simulink model "RP_VEX_V5_Gamepad_Control"  (R2019b)
settings: Solver=VariableStepAuto  StartTime=0.0  StopTime=inf  FixedStep=0.01  RelTol=1e-3  EnableMultiTasking=on
InitFcn:
  | RPInit
model workspace (MAT data in the model file):
  mapForSim.obsMap = [0 0 0 0 0 0 0 0 0 0 0 0 ... (25000 elements, 200x125)]
  mapForSim.scaleFactor = 25
  mapForSim.simMap = robotics.BinaryOccupancyGrid
  mapForSim.simMap.Grid = [1 1 1 1 1 1 1 1 1 1 1 1 ... (25000 elements, 200x125)]
  mapForSim.simMap.LayerName = "binaryLayer"
  mapForSim.simMap.Index = matlabshared.autonomous.internal.CircularBufferIndex
  mapForSim.simMap.Index.Head = [1 1]
  mapForSim.simMap.Index.Size = [200 125]
  mapForSim.simMap.Index.NewRegions = [0 0 0 0]
  mapForSim.simMap.Index.DropEntireMap = 0
  mapForSim.simMap.Index.DropTwoRegions = [0 0]
  mapForSim.simMap.Buffer = matlabshared.autonomous.internal.CircularBuffer
  mapForSim.simMap.Buffer.ConstVal = 0
  mapForSim.simMap.Buffer.DataType = 'logical'
  mapForSim.simMap.Buffer.Index = matlabshared.autonomous.internal.CircularBufferIndex
  mapForSim.simMap.Buffer.Index.Head = [1 1]
  mapForSim.simMap.Buffer.Index.Size = [200 125]
  mapForSim.simMap.Buffer.Index.NewRegions = [0 0 0 0]
  mapForSim.simMap.Buffer.Index.DropEntireMap = 0
  mapForSim.simMap.Buffer.Index.DropTwoRegions = [0 0]
  mapForSim.simMap.Buffer.Buffer = [1 1 1 1 1 1 1 1 1 1 1 1 ... (25000 elements, 200x125)]
  mapForSim.simMap.DefaultValueInternal = 0
  mapForSim.simMap.HasParent = 0
  mapForSim.simMap.Resolution = 25
  mapForSim.simMap.GridSize = [200 125]
  mapForSim.simMap.GridOriginInLocal = [0 0]
  mapForSim.simMap.LocalOriginInWorld = [0 0]
  mapForSim.simMap.Width = 5
  mapForSim.simMap.Height = 8
  mapForSim.simMap.LocalOriginInWorldInternal = [0 0]
  occGrid = robotics.BinaryOccupancyGrid
  occGrid.Grid = [1 1 1 1 1 1 1 1 1 1 1 1 ... (25000 elements, 200x125)]
  occGrid.LayerName = "binaryLayer"
  occGrid.Index = matlabshared.autonomous.internal.CircularBufferIndex
  occGrid.Index.Head = [1 1]
  occGrid.Index.Size = [200 125]
  occGrid.Index.NewRegions = [0 0 0 0]
  occGrid.Index.DropEntireMap = 0
  occGrid.Index.DropTwoRegions = [0 0]
  occGrid.Buffer = matlabshared.autonomous.internal.CircularBuffer
  occGrid.Buffer.ConstVal = 0
  occGrid.Buffer.DataType = 'logical'
  occGrid.Buffer.Index = matlabshared.autonomous.internal.CircularBufferIndex
  occGrid.Buffer.Index.Head = [1 1]
  occGrid.Buffer.Index.Size = [200 125]
  occGrid.Buffer.Index.NewRegions = [0 0 0 0]
  occGrid.Buffer.Index.DropEntireMap = 0
  occGrid.Buffer.Index.DropTwoRegions = [0 0]
  occGrid.Buffer.Buffer = [1 1 1 1 1 1 1 1 1 1 1 1 ... (25000 elements, 200x125)]
  occGrid.DefaultValueInternal = 0
  occGrid.HasParent = 0
  occGrid.Resolution = 25
  occGrid.GridSize = [200 125]
  occGrid.GridOriginInLocal = [0 0]
  occGrid.LocalOriginInWorld = [0 0]
  occGrid.Width = 5
  occGrid.Height = 8
  occGrid.LocalOriginInWorldInternal = [0 0]
undefined symbols (not defined in the file): FloorSurface, Ref, RobotSurface, X, Y, Z
libraries: sm_lib x21, RP_Simulator_Components x12, nesl_utility x11, simulink x3, vexv5lib x3, RoboticsPlayground x2, vexcommonlib x1, vrlib x1
(part 1 of 2)
settings Model: EnablePacing=on  ExtModeTrigDuration=25  Creator=scastro  LastModifiedBy=josea
settings SolverCC: AlgebraicLoopSolver=LineSearch
settings DataIOCC: LimitDataPoints=on  ReturnWorkspaceOutputs=off
settings OptimizationCC: PassReuseOutputArgsAs=Individual arguments  MaxStackSize=64  EfficientTunableParamExpr=on
settings DebuggingCC: ParameterTunabilityLossMsg=error  UnconnectedLineMsg=none  AllowSymbolicDim=off  SFUnexpectedBacktrackingDiag=warning  SFNoUnconditionalDefaultTransitionDiag=warning  SFExecutionAtInitializationDiag=none  ArithmeticOperatorsInVariantConditions=warning
settings HardwareCC: ProdBitPerPointer=32  ProdBitPerSizeT=32  ProdBitPerPtrDiffT=32  ProdLargestAtomicInteger=Long  ProdLargestAtomicFloat=Double  ProdWordSize=32  ProdHWDeviceType=ARM Compatible->ARM Cortex
settings SFSimCC: SimUseLocalCustomCode=off  MATLABDynamicMemAlloc=off  CustomCodeUndefinedFunction=UseInterfaceOnly
settings RTWCC: SystemTargetFile=ert.tlc  HardwareBoard=VEX V5 Robot Brain  TLCOptions="-aInlineSetEventsForThisBaseRateFcn=TLC_FALSE -aSuppressMultiTaskScheduler=TLC_FALSE  -aRateBasedStepFcn=0"  TemplateMakefile=ert_default_tmf  GenerateReport=on  RTWUseLocalCustomCode=off  Toolchain=GNU Tools for ARM Embedded Processors  IncludeHyperlinkInReport=on  LaunchReport=on  GenerateTraceInfo=on  GenerateTraceReport=on  GenerateTraceReportSl=on  GenerateTraceReportSf=on  GenerateTraceReportEml=on
settings CodeAppCC: ForceParamTrailComments=on  IgnoreCustomStorageClasses=off  OperatorAnnotations=on  SimulinkDataObjDesc=on  SFDataObjDesc=on  InsertBlockDesc=on
settings ERTTargetCC: ExtModeStaticAllocSize=2048
settings ConfigComp: CovMetricSettings=dw  CovHtmlReporting=on  CovSaveCumulativeToWorkspaceVar=on  CovSaveSingleToWorkspaceVar=on  CovExternalEMLEnable=off  CovSFcnEnable=off
settings SimscapeCC: SimscapeNominalValues="[{\"value\":\"10\",\"unit\":\"V\"},{\"value\":\"1\",\"unit\":\"A\"},{\"value\":\"10\",\"unit\":\"N*m\"},{\"value\":\"10\",\"unit\":\"bar\"},{\"value\":\"100\",\"unit\":\"kJ/kg\"},{\"value\":\"1\",\"unit\":\"kW\"},{\"value\":\"300\",\"unit\":\"K\"},{\"value\":\"100\",\"unit\":\"cm^3/s\"},{\"value\":\"1\",\"unit\":\"kN\"},{\"value\":\"1\",\"unit\":\"g/cm^3\"},{\"value\":\"1\",\"unit\":\"l\"},{\"value\":\"1\",\"unit\":\"cm^2\"},{\"value\":\"60\",\"unit\":\"Hz\"}]"  SimscapeLogDataHistory=10000
settings ConfigurationSet: Description=SimMechanics 2G
settings DiagnosticsConfigSet: SimMechanicsRigidlyBoundBlock=none
settings ExplorerConfigSet: InternalSimMechanicsExplorerSettings="<ExplorerConfiguration><canonicalview>default</canonicalview><AnimationSetting><BasePlaybackSpeed>1.0</BasePlaybackSpeed><PlaybackSpeedFactor>1.0</PlaybackSpeedFactor></AnimationSetting><TilePanel><TileInfo><Tiles Columns=\"2\" Count=\"3\" Rows=\"2\"><Column Weight=\"0.5\"/><Column Weight=\"0.5\"/><Row Weight=\"0.5558\"/><Row Weight=\"0.4442\"/><Tile Height=\"1\" Width=\"2\" X=\"0\" Y=\"0\"/><Tile Height=\"1\" Width=\"1\" X=\"0\" Y=\"1\"/><Tile Height=\"1\" Width=\"1\" X=\"1\" Y=\"1\"/></Tiles></TileInfo><SceneInfo><SceneViewer><BGColor><R>0.60000002384185791</R><G>0.60000002384185791</G><B>0.60000002384185791</B></BGColor><Camera><DoPerspective>off</DoPerspective><Position><X>3.77812343469301437</X><Y>-3.77812335288872925</Y><Z>3.7781233369241094</Z></Position><Center><X>-2.07139932301910341e-08</X><Y>1.02518278512960765e-07</Y><Z>-1.18482898008922e-07</Z></Center><Up><X>-0.408248290463863073</X><Y>0.408248290463863073</Y><Z>0.816496580927726145</Z></Up><ViewLimDist>1</ViewLimDist><YLim>2.86778095960617074</YLim><XLim>6.75102172519388599</XLim></Camera></SceneViewer><SceneViewer><BGColor><R>0.60000002384185791</R><G>0.60000002384185791</G><B>0.60000002384185791</B></BGColor><Camera><DoPerspective>on</DoPerspective><Position><X>0.025687663764123736</X><Y>0.399310018201750161</Y><Z>0.453907703599162216</Z></Position><Center><X>0.541332794341274459</X><Y>-0.386267680610761999</Y><Z>0.111887560273493503</Z></Center><Up><X>0.187679478974392022</X><Y>-0.285926899071094254</Y><Z>0.939692620785908428</Z></Up><ViewLimDist>1</ViewLimDist><YLim>0.466307658154998583</YLim><XLim>0.683848507606772515</XLim></Camera></SceneViewer><SceneViewer><BGColor><R>0.60000002384185791</R><G>0.60000002384185791</G><B>0.60000002384185791</B></BGColor><Camera><DoPerspective>off</DoPerspective><Position><X>-0.018234885227883621</X><Y>-0.0300165861003731764</Y><Z>37.6782594368875863</Z></Position><Center><X>-0.018234885227883621</X><Y>-0.0300165861003731764</Y><Z>0.069999846435872648</Z></Center><Up><X>0</X><Y>1</Y><Z>-0</Z></Up><ViewLimDist>1</ViewLimDist><YLim>5.44437616630040022</YLim><XLim>7.98427486888250648</XLim></Camera></SceneViewer></SceneInfo></TilePanel><MechEditorPanel><Cameras><Camera><Id>Camera1</Id><Value><Name>RobotView</Name><NativeCamera><PositionTrackingFeature>Obstacle_Environment.Robot.Body.RobotCamera.F</PositionTrackingFeature><CenterTrackingFeature>Obstacle_Environment.Robot.Body.RobotCamera.F</CenterTrackingFeature><UpVectorTrackingFeature>Obstacle_Environment.Robot.Body.RobotCamera.F</UpVectorTrackingFeature><CenterTrackingOrigin>off</CenterTrackingOrigin><CenterTrackingDirection>+X</CenterTrackingDirection><UpVectorTrackingDirection>+Z</UpVectorTrackingDirection></NativeCamera></Value></Camera></Cameras><GfxPanelCameraMap><MapElement CameraMLId=\"Camera1\" GfxPanelIndex=\"1\"/></GfxPanelCameraMap><VideoCreator><PlaybackSpeedRatio>1.0</PlaybackSpeedRatio><FrameRate>30</FrameRate><VideoFormat>Motion JPEG AVI</VideoFormat><FrameSize>auto</FrameSize></VideoCreator></MechEditorPanel></ExplorerConfiguration>"

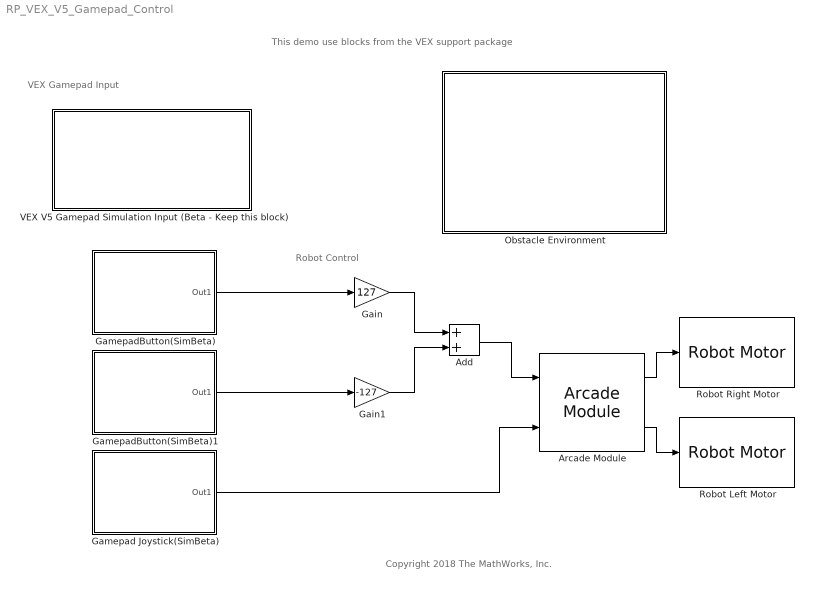
== system RP_VEX_V5_Gamepad_Control ==
  note: VEX Gamepad Input
  note: Robot Control
  note: Copyright 2018 The MathWorks, Inc.
  note: This demo use blocks from the VEX support package
  Add : Sum
  Arcade Module : vexcommonlib/Arcade Module  BlockPlatform=vexarmcortex
      settings: SourceProductName=Simulink Coder Support Package for ARM Cortex-based VEX Microcontroller  SourceProductBaseCode=EC_VEX_MICRO
  Gain : Gain  Gain=127
  Gain1 : Gain  Gain=-127
  Gamepad Joystick(SimBeta) : Subsystem  mask(Gamepad Joystick (Simulation Beta)){joystickType=Master, chan=1, SampleTime=0.02}
      mask prompts: joystickType "Joystick Type:"; chan "Analog Channel (1 to 4):"; SampleTime "Sample time:"
      mask help:
      | Read the value from one of the control axis of the analog joysticks on the VEX® gamepad(V5 controller).
      |
      | The output ranges from -128 to 127 and 0 indicates that the joystick has not been displaced.
      |
      | Use Gamepad Type to configure the gamepad to operate in Master or Partner mode.
      |
      | Use the Analog Channel drop-down to specify the control axis of the joystick on the VEX® gamepad from which you would like to read an analog signal. The Analog Channel number must match the labels on the gamepad.
      mask init:
      | chan = get_param(gcb, 'chan');
      | joyIdStr = get_param(gcb,'joystickType');
      | if strcmp(joyIdStr,'Partner')
      |     joyId='2';
      | else
      |     joyId='1';
      | end
      | 
      | set_param([gcb '/GamepadJoysticks'],'GoToTag',['simGamepadJoysticks_' joyId]);
      | 
      | if chan == '2' 
      |     md = 'icon=imread(fullfile(codertarget.vexv5.internal.getSpPkgRootDir, ''resources'', ''JoystickAnalog2.png''));icon(1:350,1:772,:)=imread(''vexv5GamepadSimInput.PNG'');image(icon)';
      |     set_param([gcb '/Channel'],'Value',chan);
      | elseif chan == '1'
      |     md = 'icon=imread(fullfile(codertarget.vexv5.internal.getSpPkgRootDir, ''resources'', ''JoystickAnalog1.png''));icon(1:350,1:772,:)=imread(''vexv5GamepadSimInput.PNG'');image(icon)';   
      |     set_param([gcb '/Channel'],'Value',chan);
      | elseif chan == '4'
      |     md = 'icon=imread(fullfile(codertarget.vexv5.internal.getSpPkgRootDir, ''resources'', ''JoystickAnalog4.png''));icon(1:350,1:772,:)=imread(''vexv5GamepadSimInput.PNG'');image(icon)';   
      |     set_param([gcb '/Channel'],'Value',chan);
      | elseif chan == '3'
      |     md = 'icon=imread(fullfile(codertarget.vexv5.internal.getSpPkgRootDir, ''resources'', ''JoystickAnalog3.png''));icon(1:350,1:772,:)=imread(''vexv5GamepadSimInput.PNG'');image(icon)';    
      |     set_param([gcb '/Channel'],'Value',chan);
      | end
      | blPosition = get_param(gcb, 'Position');
      | textSize = get_param(gcb, 'fontSize');
      | if textSize==-1
      |     textSize = get_param(bdroot, 'DefaultBlockFontSize');
      | end
      | md = codertarget.vexv5.internal.writeVEXOnMask(gcb, md);
      | set_param(gcb, 'MaskDisplay', md);
      mask TypeOptions joystickType: Gamepad Joystick/joystickType
      mask TypeOptions chan: Gamepad Joystick/chan
      mask TypeOptions SampleTime: Gamepad Joystick/SampleTime
      mask Display:
      | icon=imread(fullfile(codertarget.vexv5.internal.getSpPkgRootDir, 'resources', 'JoystickAnalog1.png'));icon(1:350,1:772,:)=imread('vexv5GamepadSimInput.PNG');image(icon)
      | patch([0.65, 0.65, 1, 1], [0.85, 1, 1, 0.85], [1, 1, 1]);
      | color('blue');
      | text(1, 1, 'VEX V5', 'horizontalAlignment', 'right', 'verticalAlignment','top');
  GamepadButton(SimBeta) : Subsystem  mask(Gamepad Button (Simulation Beta)){joystickType=Master, chan=UP, SampleTime=0.02}
      mask prompts: joystickType "Joystick Type:"; chan "Button:"; SampleTime "Sample time:"
      mask help:
      | Read the logical value of the selected button from the VEX® gamepad(V5 controller).
      |
      | The  output is 1 while the button is in pressed state and 0 while the button is in release state.
      |
      | Use Gamepad Type to configure the gamepad to operate in Master or Partner mode.
      | Use the Button drop-down to specify the button on the VEX® gamepad from which you would like to read a digital signal. The Button must match the labels on the gamepad.
      mask init:
      | chan = get_param(gcb, 'chan');
      | joyIdStr = get_param(gcb,'joystickType');
      | if strcmp(joyIdStr,'Partner')
      |     joyId='2';
      | else
      |     joyId='1';
      | end
      | set_param([gcb '/GamepadButtons'],'GoToTag',['simGamepadButtons_' joyId]);
      | 
      | if strcmp(chan,'L2') 
      |     md = 'icon=imread(fullfile(codertarget.vexv5.internal.getSpPkgRootDir, ''resources'', ''JoystickDigitalButton_L2.png''));icon(1:31,1:60,:)=imread(''vexv5GamepadSimInput2.PNG'');image(icon)';
      |     set_param([gcb '/Channel'],'Value','10');
      | elseif strcmp(chan,'L1') 
      |     md = 'icon=imread(fullfile(codertarget.vexv5.internal.getSpPkgRootDir, ''resources'', ''JoystickDigitalButton_L1.png''));icon(1:31,1:60,:)=imread(''vexv5GamepadSimInput2.PNG'');image(icon)';
      |     set_param([gcb '/Channel'],'Value','9');
      | elseif strcmp(chan,'R2') 
      |     md = 'icon=imread(fullfile(codertarget.vexv5.internal.getSpPkgRootDir, ''resources'', ''JoystickDigitalButton_R2.png''));icon(1:31,1:60,:)=imread(''vexv5GamepadSimInput2.PNG'');image(icon)';
      |     set_param([gcb '/Channel'],'Value','12');
      | elseif strcmp(chan,'R1') 
      |     md = 'icon=imread(fullfile(codertarget.vexv5.internal.getSpPkgRootDir, ''resources'', ''JoystickDigitalButton_R1.png''));icon(1:31,1:60,:)=imread(''vexv5GamepadSimInput2.PNG'');image(icon)';
      |     set_param([gcb '/Channel'],'Value','11');
      | elseif strcmp(chan,'DOWN') 
      |      md = 'icon=imread(fullfile(codertarget.vexv5.internal.getSpPkgRootDir, ''resources'', ''JoystickDigitalDown.png''));icon(1:31,1:60,:)=imread(''vexv5GamepadSimInput2.PNG'');image(icon)';
      |      set_param([gcb '/Channel'],'Value','2');
      | elseif strcmp(chan,'UP') 
      |     md = 'icon=imread(fullfile(codertarget.vexv5.internal.getSpPkgRootDir, ''resources'', ''JoystickDigitalUp.png''));icon(1:31,1:60,:)=imread(''vexv5GamepadSimInput2.PNG'');image(icon)';
      |     set_param([gcb '/Channel'],'Value','1');
      | elseif strcmp(chan,'LEFT') 
      |     md = 'icon=imread(fullfile(codertarget.vexv5.internal.getSpPkgRootDir, ''resources'', ''JoystickDigitalLeft.png''));icon(1:31,1:60,:)=imread(''vexv5GamepadSimInput2.PNG'');image(icon)';
      |     set_param([gcb '/Channel'],'Value','3');
      | elseif strcmp(chan,'RIGHT') 
      |     md = 'icon=imread(fullfile(codertarget.vexv5.internal.getSpPkgRootDir, ''resources'', ''JoystickDigitalRight.png''));icon(1:31,1:60,:)=imread(''vexv5GamepadSimInput2.PNG'');image(icon)';
      |     set_param([gcb '/Channel'],'Value','4');
      | elseif chan == 'B' 
      |     md = 'icon=imread(fullfile(codertarget.vexv5.internal.getSpPkgRootDir, ''resources'', ''JoystickDigitalButton_B.png''));icon(1:31,1:60,:)=imread(''vexv5GamepadSimInput2.PNG'');image(icon)';
      |     set_param([gcb '/Channel'],'Value','6');
      | elseif chan == 'X' 
      |     md = 'icon=imread(fullfile(codertarget.vexv5.internal.getSpPkgRootDir, ''resources'', ''JoystickDigitalButton_X.png''));icon(1:31,1:60,:)=imread(''vexv5GamepadSimInput2.PNG'');image(icon)';
      |     set_param([gcb '/Channel'],'Value','7');
      | elseif chan == 'Y' 
      |     md = 'icon=imread(fullfile(codertarget.vexv5.internal.getSpPkgRootDir, ''resources'', ''JoystickDigitalButton_Y.png''));icon(1:31,1:60,:)=imread(''vexv5GamepadSimInput2.PNG'');image(icon)';
      |     set_param([gcb '/Channel'],'Value','8');
      | elseif chan == 'A' 
      |     md = 'icon=imread(fullfile(codertarget.vexv5.internal.getSpPkgRootDir, ''resources'', ''JoystickDigitalButton_A.png''));icon(1:31,1:60,:)=imread(''vexv5GamepadSimInput2.PNG'');image(icon)';
      |     set_param([gcb '/Channel'],'Value','5');
      | end
      | 
      | md = codertarget.vexv5.internal.writeVEXOnMask(gcb, md);
      | set_param(gcb, 'MaskDisplay', md);
      mask TypeOptions joystickType: Gamepad Button/joystickType
      mask TypeOptions chan: Gamepad Button/chan
      mask TypeOptions SampleTime: Gamepad Button/SampleTime
      mask Display:
      | icon=imread(fullfile(codertarget.vexv5.internal.getSpPkgRootDir, 'resources', 'JoystickDigitalUp.png'));icon(1:31,1:60,:)=imread('vexv5GamepadSimInput2.PNG');image(icon)
      | patch([0.65, 0.65, 1, 1], [0.85, 1, 1, 0.85], [1, 1, 1]);
      | color('blue');
      | text(1, 1, 'VEX V5', 'horizontalAlignment', 'right', 'verticalAlignment','top');
  GamepadButton(SimBeta)1 : Subsystem  mask(Gamepad Button (Simulation Beta)){joystickType=Master, chan=DOWN, SampleTime=0.02}
      mask prompts: joystickType "Joystick Type:"; chan "Button:"; SampleTime "Sample time:"
      mask help:
      | Read the logical value of the selected button from the VEX® gamepad(V5 controller).
      |
      | The  output is 1 while the button is in pressed state and 0 while the button is in release state.
      |
      | Use Gamepad Type to configure the gamepad to operate in Master or Partner mode.
      | Use the Button drop-down to specify the button on the VEX® gamepad from which you would like to read a digital signal. The Button must match the labels on the gamepad.
      mask init: same as RP_VEX_V5_Gamepad_Control/GamepadButton(SimBeta)
      mask TypeOptions joystickType: Gamepad Button/joystickType
      mask TypeOptions chan: Gamepad Button/chan
      mask TypeOptions SampleTime: Gamepad Button/SampleTime
      mask Display:
      | icon=imread(fullfile(codertarget.vexv5.internal.getSpPkgRootDir, 'resources', 'JoystickDigitalDown.png'));icon(1:31,1:60,:)=imread('vexv5GamepadSimInput2.PNG');image(icon)
      | patch([0.65, 0.65, 1, 1], [0.85, 1, 1, 0.85], [1, 1, 1]);
      | color('blue');
      | text(1, 1, 'VEX V5', 'horizontalAlignment', 'right', 'verticalAlignment','top');
  Obstacle Environment : Subsystem  mask(RP Obstacle Environment){obs1=on, obsPose1=[0.14251      3.2953], obsWidth1=4.0293, obsLength1=0.31625, obs2=on, obsPose2=[1.8233    -0.44119], obsWidth2=0.24597, obsLength2=5.7042, obs3=on, obsPose3=[-0.33772     -3.1938], obsWidth3=3.3734, obsLength3=0.55051, obs4=on, obsPose4=[-0.43729    -0.97413], obsWidth4=3.1274, obsLength4=0.37482, obs5=off, obsPose5=[1.6535    -0.67545], obsWidth5=0.39824, obsLength5=0.71449, obs6=off, obsPose6=[3.1293     -1.6301], obsWidth6=0.60322, obsLength6=0.47438, obs7=off, obsPose7=[2 2], obsWidth7=0.8, obsLength7=0.4, obs8=off, obsPose8=[2 2], obsWidth8=0.8, obsLength8=0.4, obs9=off, obsPose9=[2 2], obsWidth9=0.8, obsLength9=0.4, obs10=off, obsPose10=[2 2], obsWidth10=0.8, obsLength10=0.4, arenaLength=5, arenaWidth=8, robotId=1, wheelBase=0.5, wheelRadius=0.1, robotColor=[0 0 0.5], startPose=[-1.4 0]}
      mask prompts: obs1 "Enable"; obsPose1 "Position X Y [m]"; obsWidth1 "Width [m]"; obsLength1 "Length [m]"; obs2 "Enable"; obsPose2 "Position X Y [m]"; obsWidth2 "Width [m]"; obsLength2 "Length [m]"; obs3 "Enable"; obsPose3 "Position X Y [m]"; obsWidth3 "Width [m]"; obsLength3 "Length [m]"; obs4 "Enable"; obsPose4 "Position X Y [m]"; obsWidth4 "Width [m]"; obsLength4 "Length [m]"; obs5 "Enable"; obsPose5 "Position X Y [m]"; obsWidth5 "Width [m]"; obsLength5 "Length [m]"; obs6 "Enable"; obsPose6 "Position X Y [m]"; obsWidth6 "Width [m]"; obsLength6 "Length [m]"; obs7 "Enable"; obsPose7 "Position X Y [m]"; obsWidth7 "Width [m]"; obsLength7 "Length [m]"; obs8 "Enable"; obsPose8 "Position X Y [m]"; obsWidth8 "Width [m]"; obsLength8 "Length [m]"; obs9 "Enable"; obsPose9 "Position X Y [m]"; obsWidth9 "Width [m]"; obsLength9 "Length [m]"; obs10 "Enable"; obsPose10 "Position X Y [m]"; obsWidth10 "Width [m]"; obsLength10 "Length [m]"; arenaLength "Length [m]"; arenaWidth "Width [m]"; robotId "Robot ID"; wheelBase "Distance between wheels [m]"; wheelRadius "Wheel radius [m]"; robotColor "Color [R G B]"; startPose "Initial Position X Y [m]"
      mask help:
      | This block contains a virtual environment for a single robot to interact with walls, obstacles and objects. Sensors implemented in the Robotics Playground library can be used to obtain environment information and actuators to interact with the robot behavior.
      |
      | Motor mapping for the robot is as follows:
      |
      | Motor 1 -> Left wheel motor torque
      | Motor 2 -> Right wheel motor torque
      settings: CopyFcn=|
      | set_param(gcs,'InitFcn','RPInit');
      | set_param(gcs,'Solver','ode23t');
      | set_param(gcs, 'EnablePacing', 'on')
      | set_param(gcs, 'PacingRate', 1)
      mask Help: web('obstacle_arena.htm')
      mask Callback obs1: commentObstacles(gcb)
      mask Callback obs2: commentObstacles(gcb)
      mask Callback obs3: commentObstacles(gcb)
      mask Callback obs4: commentObstacles(gcb)
      mask Callback obs5: commentObstacles(gcb)
      mask Callback obs6: commentObstacles(gcb)
      mask Callback obs7: commentObstacles(gcb)
      mask Callback obs8: commentObstacles(gcb)
      mask Callback obs9: commentObstacles(gcb)
      mask Callback obs10: commentObstacles(gcb)
      mask DialogControl obsT Prompt: Obstacle settings
      mask DialogControl Container19 Prompt: Set Obstacles Interactively
      mask DialogControl Control2 Prompt: Set Obstacles
      mask DialogControl Control2 Callback: setObstaclesUI(gcb)
      mask DialogControl Control3 Prompt: Disable all obstacles
      mask DialogControl Control3 Callback: disableObstacles(gcb)
      mask DialogControl Container21 Prompt: Obstacle Details
      mask DialogControl obsc1 Prompt: Obstacle 1
      mask DialogControl obsc2 Prompt: Obstacle 2
      mask DialogControl obsc3 Prompt: Obstacle 3
      mask DialogControl obsc4 Prompt: Obstacle 4
      mask DialogControl obsc5 Prompt: Obstacle 5
      mask DialogControl obsc6 Prompt: Obstacle 6
      mask DialogControl obsc7 Prompt: Obstacle 7
      mask DialogControl obsc8 Prompt: Obstacle 8
      mask DialogControl obsc9 Prompt: Obstacle 9
      mask DialogControl obsc10 Prompt: Obstacle 10
      mask DialogControl Container6 Prompt: Arena settings
      mask DialogControl Container4 Prompt: Robot settings
      mask Display:
      | color('white');
      | plot([100,100,100,100]*1,[100,100,100,100]*1);
      | plot([100,100,100,100]*0,[100,100,100,100]*0);
      | image('ObstacleEnv.PNG')
      | color('blue');
      | id=eval(get_param(gcb,'robotId'));
      | text(99, 92, ['Robot ID: ' num2str(id)], 'horizontalAlignment', 'right');
  Robot Left Motor : RoboticsPlayground/Basic Sensors and Actuators/Robot Motor  robotId=1  motorChoice=1
      settings: SourceProductName=Robotics Playground
  Robot Right Motor : RoboticsPlayground/Basic Sensors and Actuators/Robot Motor  robotId=1  motorChoice=2
      settings: SourceProductName=Robotics Playground
  VEX V5 Gamepad Simulation Input (Beta - Keep this block) : Subsystem  mask(VEX V5 Gamepad Simulation Input){gamepadChoice=1- Master}
      mask prompts: gamepadChoice "Gamepad Selection"
      mask help: This blocks uses the input from the VEX V5 Gamepad for desktop simulations. A V5 gamepad must be connected directly to the computer using a USB cable.
      mask init:
      | joyIdStr = get_param(gcb,'gamepadChoice');
      | if strcmp(joyIdStr,'2- Partner')
      |     joyId='2';
      | else
      |     joyId='1';
      | end
      | set_param([gcb '/Joystick Input'],'joyid',joyId);
      | set_param([gcb '/GamepadJoysticks'],'GoToTag',['simGamepadJoysticks_' joyId]);
      | set_param([gcb '/GamepadButtons'],'GoToTag',['simGamepadButtons_' joyId]);
      mask TypeOptions gamepadChoice: 1- Master | 2- Partner
      mask Display: image('vexv5GamepadSimInput.PNG')
  wires:
  Arcade Module/1 -> Robot Right Motor/1
  Arcade Module/2 -> Robot Left Motor/1
  Add/1 -> Arcade Module/1
  Gamepad Joystick(SimBeta)/1(Out1) -> Arcade Module/2
  GamepadButton(SimBeta)/1(Out1) -> Gain/1
  GamepadButton(SimBeta)1/1(Out1) -> Gain1/1
  Gain/1 -> Add/1
  Gain1/1 -> Add/2

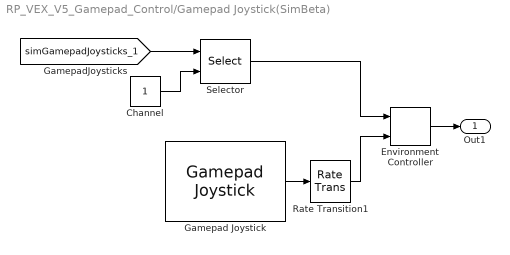
== system RP_VEX_V5_Gamepad_Control/Gamepad Joystick(SimBeta) ==
  Channel : Constant
  Environment Controller : simulink/Signal Routing/Environment Controller
      settings: SourceProductName=Simulink  SourceProductBaseCode=SL
  Gamepad Joystick : vexv5lib/Gamepad/Gamepad Joystick  joystickType=Master  chan=1  SampleTime=SampleTime
      settings: SourceProductName=Simulink Coder Support Package for VEX EDR V5 Robot Brain  SourceProductBaseCode=VEXV5
  Rate Transition1 : RateTransition
  Selector : Selector  InputPortWidth=4  IndexOptions=Index vector (port)  Indices=[1 3]  OutputSizes=1
  Out1 : Outport
  wires:
  Rate Transition1/1 -> Environment Controller/2
  Selector/1 -> Environment Controller/1
  Channel/1 -> Selector/2
  [simGamepadJoysticks_1] -> Selector/1
  Environment Controller/1 -> Out1/1
  Gamepad Joystick/1 -> Rate Transition1/1

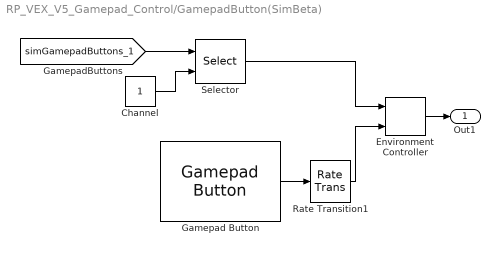
== system RP_VEX_V5_Gamepad_Control/GamepadButton(SimBeta) ==
  Channel : Constant
  Environment Controller : simulink/Signal Routing/Environment Controller
      settings: SourceProductName=Simulink  SourceProductBaseCode=SL
  Gamepad Button : vexv5lib/Gamepad/Gamepad Button  joystickType=Master  chan=UP  SampleTime=SampleTime
      settings: SourceProductName=Simulink Coder Support Package for VEX EDR V5 Robot Brain  SourceProductBaseCode=VEXV5
  Rate Transition1 : RateTransition
  Selector : Selector  InputPortWidth=12  IndexOptions=Index vector (port)  Indices=[1 3]  OutputSizes=1
  Out1 : Outport
  wires:
  Rate Transition1/1 -> Environment Controller/2
  Gamepad Button/1 -> Rate Transition1/1
  Environment Controller/1 -> Out1/1
  [simGamepadButtons_1] -> Selector/1
  Channel/1 -> Selector/2
  Selector/1 -> Environment Controller/1

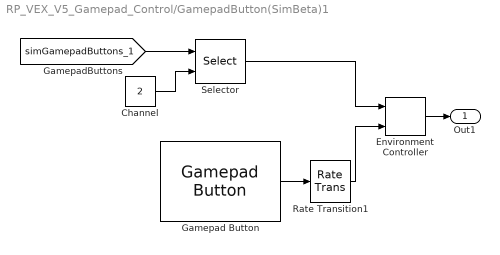
== system RP_VEX_V5_Gamepad_Control/GamepadButton(SimBeta)1 ==
  Channel : Constant  Value=2
  Environment Controller : simulink/Signal Routing/Environment Controller
      settings: SourceProductName=Simulink  SourceProductBaseCode=SL
  Gamepad Button : vexv5lib/Gamepad/Gamepad Button  joystickType=Master  chan=DOWN  SampleTime=SampleTime
      settings: SourceProductName=Simulink Coder Support Package for VEX EDR V5 Robot Brain  SourceProductBaseCode=VEXV5
  Rate Transition1 : RateTransition
  Selector : Selector  InputPortWidth=12  IndexOptions=Index vector (port)  Indices=[1 3]  OutputSizes=1
  Out1 : Outport
  wires:
  Selector/1 -> Environment Controller/1
  Channel/1 -> Selector/2
  [simGamepadButtons_1] -> Selector/1
  Environment Controller/1 -> Out1/1
  Gamepad Button/1 -> Rate Transition1/1
  Rate Transition1/1 -> Environment Controller/2

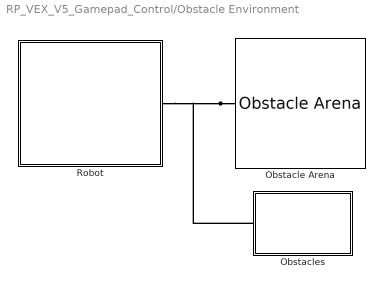
== system RP_VEX_V5_Gamepad_Control/Obstacle Environment ==
  Obstacle Arena : RP_Simulator_Components/Obstacle Arena  length=arenaLength  width=arenaWidth  robotRadius=wheelBase/2
  Obstacles : Subsystem
  Robot : Subsystem  AncestorBlock=RP_Simulator_Components/Contact Tank Robot  mask(RP Contact Tank Robot){robotId=robotId, wheelRadius=wheelRadius, wheelBase=wheelBase, wheelThickness=0.025, chassisThickness=0.05, startPose=startPose, choice=off, sensorTs=0.05, wheelMass=0.2, chassisMass=0.5, maxWheelTorque=1, floorSize=[arenaLength arenaWidth], wheelColor=[0.25 0.25 0.25], chassisColor=robotColor}
      mask prompts: robotId "Robot ID"; wheelRadius "Wheel Radius [m]"; wheelBase "Wheelbase [m]"; wheelThickness "Wheel Thickness [m]"; chassisThickness "Chassis Thickness [m]"; startPose "Start Position [m]"; choice "Reverse Start Position"; sensorTs "Sensor sample time [s]"; wheelMass "Wheel Mass [kg]"; chassisMass "Chassis Mass [kg]"; maxWheelTorque "Maximum wheel torque [N*m]"; floorSize "Floor Dimensions [m]"; wheelColor "Wheel Color"; chassisColor "Chassis Color"
      mask help:
      | This robot implements contact between the robot wheels and the floor of an arena. The stck-slip friction implemented using contact force libraries makes the robot behavior more realistic. The inputs to the robot are now motor torque, which is set using the Robotics Playground Motor blocks. The motor mappings are as follows:
      |
      | Motor 1 -> Left wheel motor torque
      | Motor 2 -> Right wheel motor torque
      mask init:
      | block=gcb;
      | ID=num2str(eval(get_param(block,'robotId')));
      | 
      | set_param([block '/motor1t'],'GotoTag',['R' ID 'motor1t']);
      | set_param([block '/motor2t'],'GotoTag',['R' ID 'motor2t']);
      | set_param([block '/motor1q'],'GotoTag',['R' ID 'motor1q']);
      | set_param([block '/motor1w'],'GotoTag',['R' ID 'motor1w']);
      | set_param([block '/motor2q'],'GotoTag',['R' ID 'motor2q']);
      | set_param([block '/motor2w'],'GotoTag',['R' ID 'motor2w']);
      | set_param([block '/xPose'],'GotoTag',['R' ID 'xPose']);
      | set_param([block '/yPose'],'GotoTag',['R' ID 'yPose']);
      | set_param([block '/tPose'],'GotoTag',['R' ID 'tPose']);
      | set_param([block '/tRate'],'GotoTag',['R' ID 'tRate']);
      | set_param([block '/tAngle'],'GotoTag',['R' ID 'tAngle']);
      | 
      | % Add sensor visuals
      | 
      | addSensors(block,eval(ID));
      mask DialogControl KinContainer Prompt: Kinematics
      mask DialogControl DynamicsContainer Prompt: Dynamics
      mask DialogControl AppearanceContainer Prompt: Appearance
      mask Display:
      | image('discRobot.PNG')
      | port_label('Rconn',1,'RP-Bus')
  connections:
  Obstacle Arena/LConn1 -- Robot/RConn1 -- Obstacles/LConn1

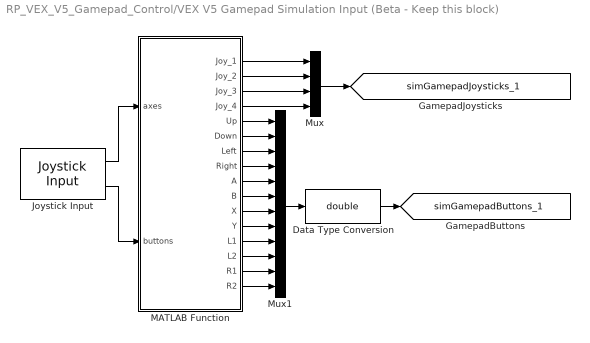
== system RP_VEX_V5_Gamepad_Control/VEX V5 Gamepad Simulation Input (Beta - Keep this block) ==
  Data Type Conversion : DataTypeConversion  OutDataTypeStr=double
  Joystick Input : vrlib/Joystick Input  joyid=1  adjustports=on  forcefeed=off
      settings: SourceProductName=Simulink
  MATLAB Function : MATLAB Function  TreatAsAtomicUnit=on
  Mux : Mux
  Mux1 : Mux  Inputs=12
  tag scope: simGamepadButtons_1=global, simGamepadJoysticks_1=global
  wires:
  Joystick Input/1 -> MATLAB Function/1(axes)
  Joystick Input/2 -> MATLAB Function/2(buttons)
  MATLAB Function/16(R2) -> Mux1/12
  MATLAB Function/15(R1) -> Mux1/11
  MATLAB Function/14(L2) -> Mux1/10
  MATLAB Function/13(L1) -> Mux1/9
  MATLAB Function/12(Y) -> Mux1/8
  MATLAB Function/11(X) -> Mux1/7
  MATLAB Function/10(B) -> Mux1/6
  MATLAB Function/9(A) -> Mux1/5
  MATLAB Function/8(Right) -> Mux1/4
  MATLAB Function/7(Left) -> Mux1/3
  MATLAB Function/6(Down) -> Mux1/2
  MATLAB Function/5(Up) -> Mux1/1
  Mux/1 -> [simGamepadJoysticks_1]
  Mux1/1 -> Data Type Conversion/1
  MATLAB Function/1(Joy_1) -> Mux/1
  MATLAB Function/2(Joy_2) -> Mux/2
  MATLAB Function/3(Joy_3) -> Mux/3
  MATLAB Function/4(Joy_4) -> Mux/4
  Data Type Conversion/1 -> [simGamepadButtons_1]

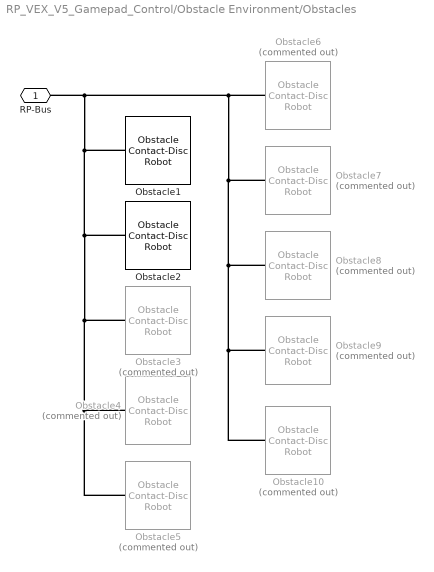
== system RP_VEX_V5_Gamepad_Control/Obstacle Environment/Obstacles ==
  Obstacle1 : RP_Simulator_Components/Obstacle Contact-Disc Robot  Pose=obsPose1  width=obsWidth1  length=obsLength1  height=0.3  color=[1.0 0.4 0.2]
  Obstacle10 : RP_Simulator_Components/Obstacle Contact-Disc Robot  Commented=on  Pose=obsPose10  width=obsWidth10  length=obsLength10  height=0.3  color=[1.0 0.4 0.2]
  Obstacle2 : RP_Simulator_Components/Obstacle Contact-Disc Robot  Pose=obsPose2  width=obsWidth2  length=obsLength2  height=0.3  color=[1.0 0.4 0.2]
  Obstacle3 : RP_Simulator_Components/Obstacle Contact-Disc Robot  Commented=on  Pose=obsPose3  width=obsWidth3  length=obsLength3  height=0.3  color=[1.0 0.4 0.2]
  Obstacle4 : RP_Simulator_Components/Obstacle Contact-Disc Robot  Commented=on  Pose=obsPose4  width=obsWidth4  length=obsLength4  height=0.3  color=[1.0 0.4 0.2]
  Obstacle5 : RP_Simulator_Components/Obstacle Contact-Disc Robot  Commented=on  Pose=obsPose5  width=obsWidth5  length=obsLength5  height=0.3  color=[1.0 0.4 0.2]
  Obstacle6 : RP_Simulator_Components/Obstacle Contact-Disc Robot  Commented=on  Pose=obsPose6  width=obsWidth6  length=obsLength6  height=0.3  color=[1.0 0.4 0.2]
  Obstacle7 : RP_Simulator_Components/Obstacle Contact-Disc Robot  Commented=on  Pose=obsPose7  width=obsWidth7  length=obsLength7  height=0.3  color=[1.0 0.4 0.2]
  Obstacle8 : RP_Simulator_Components/Obstacle Contact-Disc Robot  Commented=on  Pose=obsPose8  width=obsWidth8  length=obsLength8  height=0.3  color=[1.0 0.4 0.2]
  Obstacle9 : RP_Simulator_Components/Obstacle Contact-Disc Robot  Commented=on  Pose=obsPose9  width=obsWidth9  length=obsLength9  height=0.3  color=[1.0 0.4 0.2]
  RP-Bus : PMIOPort  Side=Left
  connections:
  RP-Bus/RConn1 -- Obstacle7/LConn1 -- Obstacle8/LConn1 -- Obstacle9/LConn1 -- Obstacle10/LConn1 -- Obstacle6/LConn1 -- Obstacle2/LConn1 -- Obstacle3/LConn1 -- Obstacle4/LConn1 -- Obstacle5/LConn1 -- Obstacle1/LConn1
